simulink model "UAV_sync_known_sim_wrong_version"  (R2018b)
settings: Solver=ode23tb  StartTime=0.0  StopTime=35
values from neighbouring files (symbols this model uses):
  C_rho = 1.225    [SC42120_UAV_Preconditions.m]
  D0 = [M0 0 0 0 0 0 ... (first row only)    [SC42120_UAV_Preconditions.m]
  D1 = [eye(3)*M1 zeros(3,3) ... (first row only)    [UAV_sync_known.m]    (also in UAV_sync_unknown.m; UAV_sync_unknown_gap.m)
  D2 = [eye(3)*M2 zeros(3,3) ... (first row only)    [UAV_sync_known.m]    (also in UAV_sync_unknown.m; UAV_sync_unknown_gap.m)
  Derivative_gain_phi = 50    [SC42120_UAV_Preconditions.m]
  Derivative_gain_psi = 50    [SC42120_UAV_Preconditions.m]
  Derivative_gain_theta = 50    [SC42120_UAV_Preconditions.m]
  Derivative_gain_x = 50    [SC42120_UAV_Preconditions.m]
  Derivative_gain_y = 50    [SC42120_UAV_Preconditions.m]
  Derivative_gain_z = 50    [SC42120_UAV_Preconditions.m]
  G = 9.80665    [SC42120_UAV_Preconditions.m]
  g0 = [0;0;-M0*G;0;0;0]    [SC42120_UAV_Preconditions.m]
  I0 = [0.02 0 -0.01 ... (first row only)    [SC42120_UAV_Preconditions.m]
  I1 = [0.1 0 -0.01 ... (first row only)    [UAV_sync_known.m]    (also in UAV_sync_unknown.m; UAV_sync_unknown_gap.m)
  I2 = 2*[0.1 0 -0.01 ... (first row only)    [UAV_sync_known.m]    (also in UAV_sync_unknown.m; UAV_sync_unknown_gap.m)
  InitWind = [0;0;0]    [SC42120_UAV_Preconditions.m]
  Kp = diag(P)    [SC42120_UAV_Preconditions.m]
  Kv = diag(V)    [SC42120_UAV_Preconditions.m]
  M0 = 10    [SC42120_UAV_Preconditions.m]
  M1 = 20    [UAV_sync_known.m]    (also in UAV_sync_unknown.m; UAV_sync_unknown_gap.m)
  M2 = 30    [UAV_sync_known.m]    (also in UAV_sync_unknown.m; UAV_sync_unknown_gap.m)
  Proportional_phi = 50    [SC42120_UAV_Preconditions.m]
  Proportional_psi = 50    [SC42120_UAV_Preconditions.m]
  Proportional_theta = 50    [SC42120_UAV_Preconditions.m]
  Proportional_x = 50    [SC42120_UAV_Preconditions.m]
  Proportional_y = 50    [SC42120_UAV_Preconditions.m]
  Proportional_z = 50    [SC42120_UAV_Preconditions.m]
undefined symbols (not defined in the file or in its folder): Aero, APlane, Bxl, C, Ctr, deg, DiscIntNeverNeededParam, F, Guid, Init, Light, MIL, Path, rad, s, Trim, Utility
libraries: aerolibconvert2 x37, simulink x15, dspsigops x7, shared6dof x4, aerolibasang x4, sharedutil x4, simulink_extras x3, aerolibadyn x1, aerolibtransform2 x1, aerolibwind2 x1
(part 5 of 6)

== system UAV_sync_known_sim_wrong_version/Node 0/VF Approach/BIXLER DYNAMICS/Vehicle Airframe/Aerodynamics/Forces//Moments ==
  note: From stability frame to body frame
  CD : Inport
  Cy : Inport  Port=2
  CL : Inport  Port=3
  Cl : Inport  Port=4
  Cm : Inport  Port=5
  Cn : Inport  Port=6
  DerCond : Inport  Port=7
  "Aerodynamic Forces and Moments " : aerolibadyn/Aerodynamic Forces and Moments   inputAxes=Body  outputForceAxes=Body  outputMomentAxes=Body  S=Bxl.S  b=Bxl.c  cbar=Bxl.b
      settings: SourceProductName=Aerospace Blockset
  Bus Selector : BusSelector  OutputSignals=qbar
  Constant : Constant  Value=Bxl.COG
  Demux : Demux  Outputs=3
  From wind to body : Math  Operator=transpose  SaturateOnIntegerOverflow=on
  Gain2 : Gain  Gain=-1
  Gain3 : Gain  Gain=-1
  Manual Switch : ManualSwitch  CurrentSetting=0
  Mux : Mux  Inputs=6
  Mux1 : Mux  Inputs=3
  Mux3 : Mux  Inputs=2
  Product : Product  Inputs=**  Multiplication=Matrix(*)
  Rotation Matrix Body to Wind : aerolibtransform2/Direction Cosine Matrix Body to Wind
      settings: SourceProductName=Aerospace Blockset  SourceProductBaseCode=AE
  beta : Constant  Value=0
  neglect center of gravity and center of pressure effects : Constant  Value=[0 0 0]
  Fxyz : Outport
  Mlmn : Outport  Port=2
  wires:
  Demux/1 -> Mux/1  "Cx"
  Demux/3 -> Mux/3  "Cz"
  Mux/1 -> "Aerodynamic Forces and Moments "/1
  Cn/1 -> Mux/6
  CD/1 -> Gain2/1
  Cl/1 -> Mux/4
  Mux1/1 -> Product/2
  Constant/1 -> Manual Switch/1
  "Aerodynamic Forces and Moments "/2 -> Mlmn/1
  "Aerodynamic Forces and Moments "/1 -> Fxyz/1
  Bus Selector/1 -> "Aerodynamic Forces and Moments "/2  "<qbar>"
  DerCond/1 -> Bus Selector/1
  CL/1 -> Gain3/1
  Cm/1 -> Mux/5
  [alphaRad] -> Mux3/1
  beta/1 -> Mux3/2
  Mux3/1 -> Rotation Matrix Body to Wind/1
  Rotation Matrix Body to Wind/1 -> From wind to body/1
  Gain2/1 -> Mux1/1
  Gain3/1 -> Mux1/3
  Cy/1 -> Mux1/2
  From wind to body/1 -> Product/1
  Product/1 -> Demux/1
  Demux/2 -> Mux/2  "Cy"
  neglect center of gravity and center of pressure effects/1 -> Manual Switch/2
  Manual Switch/1 -> "Aerodynamic Forces and Moments "/4, "Aerodynamic Forces and Moments "/3

== system UAV_sync_known_sim_wrong_version/Node 0/VF Approach/BIXLER DYNAMICS/Vehicle Airframe/Propulsion/By interpolation ==
  In1 : Inport
  Prelookup : PreLookup  BreakpointsData=Aero.thrust_vect  BeginIndexSearchUsingPreviousIndexResult=on  RemoveProtectionInput=on
  Throttle interpolation : Interpolation_n-D  NumberOfTableDimensions=1  Table=Aero.thrust_force_vect  ExtrapMethod=Clip  RemoveProtectionIndex=on  InternalRulePriority=Speed
      settings: InputPortMap=u0,u1
  Out1 : Outport
  wires:
  Prelookup/1 -> Throttle interpolation/1
  Prelookup/2 -> Throttle interpolation/2
  Throttle interpolation/1 -> Out1/1
  In1/1 -> Prelookup/1

== system UAV_sync_known_sim_wrong_version/Node 0/VF Approach/BIXLER DYNAMICS/Vehicle Airframe/Propulsion/Propeller model (Bernoulli) ==
  DerCond : Inport
  Throttle : Inport  Port=2
  0.5 * C.rho * Bxl.S_prop * Bxl.rotor_thrust_coeff : Gain  Gain=0.5 * C.rho * Bxl.S_prop * Bxl.rotor_thrust_coeff
  Bus Selector : BusSelector  OutputSignals=Va
  Bxl.r_prop : Gain  Gain=Bxl.r_prop*0.5
  Math Function : Math  Operator=square  SaturateOnIntegerOverflow=on
  Math Function1 : Math  Operator=square  SaturateOnIntegerOverflow=on
  Sum : Sum  Inputs=+-
  k_motor * u + q_motor : Fcn  Expr=Bxl.k_motor * u + Bxl.q_motor
  Thrust : Outport
  wires:
  Math Function/1 -> Sum/2  "V_a^2"
  Sum/1 -> 0.5 * C.rho * Bxl.S_prop * Bxl.rotor_thrust_coeff/1
  DerCond/1 -> Bus Selector/1
  Throttle/1 -> k_motor * u + q_motor/1
  0.5 * C.rho * Bxl.S_prop * Bxl.rotor_thrust_coeff/1 -> Thrust/1  "T"
  Bxl.r_prop/1 -> Math Function1/1  "Air flow velocity after prop."
  k_motor * u + q_motor/1 -> Bxl.r_prop/1  "Prop. angular speed (Omega)"
  Math Function1/1 -> Sum/1  "(R*Ome)^2"
  Bus Selector/1 -> Math Function/1  "<Va>"

== system UAV_sync_known_sim_wrong_version/Node 0/VF Approach/PATH FOLLOWING/Orbit Path Following (Enabled Subsystem)/Chi_d/While Iterator Subsystem ==
  gamma : Inport
  chi : Inport  Port=2
  IC : Inport  Port=3
  Bias : Bias  Bias=2*pi
  Constant : Constant  Value=-pi
  Relational Operator : RelationalOperator  Operator=<  OutDataTypeStr=boolean  RndMeth=Simplest
  Sum : Sum  Inputs=|+-
  While Iterator : WhileIterator  ResetStates=reset
  gaooa_out : Outport
  wires:
  IC/1 -> While Iterator/2
  gamma/1 -> Bias/1, Sum/1
  chi/1 -> Sum/2
  Sum/1 -> Relational Operator/1
  Constant/1 -> Relational Operator/2
  Relational Operator/1 -> While Iterator/1
  Bias/1 -> gaooa_out/1

== system UAV_sync_known_sim_wrong_version/Node 0/VF Approach/PATH FOLLOWING/Orbit Path Following (Enabled Subsystem)/Chi_d/While Iterator Subsystem2 ==
  gamma : Inport
  chi : Inport  Port=2
  IC : Inport  Port=3
  Bias : Bias  Bias=2*pi
  Constant : Constant  Value=pi
  Relational Operator : RelationalOperator  Operator=>  OutDataTypeStr=boolean  RndMeth=Simplest
  Sum : Sum  Inputs=|+-
  While Iterator : WhileIterator  ResetStates=reset
  gaooa_out : Outport
  wires:
  Bias/1 -> gaooa_out/1
  Relational Operator/1 -> While Iterator/1
  Constant/1 -> Relational Operator/2
  Sum/1 -> Relational Operator/1
  chi/1 -> Sum/2
  gamma/1 -> Sum/1, Bias/1
  IC/1 -> While Iterator/2

== system UAV_sync_known_sim_wrong_version/Node 0/VF Approach/PATH FOLLOWING/Orbit Path Following (Enabled Subsystem)/Loiter Controller/Parameters Mixer ==
  Constant1 : Constant  Value=Guid.Est.alpha
  Constant6 : Constant  Value=Guid.Loiter.k
  Constant7 : Constant  Value=Guid.Loiter.kk
  Constant8 : Constant  Value=Guid.Loiter.eps
  Mux : Mux  Inputs=6
  param : Outport
  wires:
  Mux/1 -> param/1
  Constant6/1 -> Mux/1
  Constant7/1 -> Mux/2
  Constant8/1 -> Mux/3
  [R] -> Mux/4
  [j] -> Mux/5
  Constant1/1 -> Mux/6

== system UAV_sync_known_sim_wrong_version/Node 0/VF Approach/PATH FOLLOWING/Orbit Path Following (Enabled Subsystem)/Vg Estimator/Parameters Mixer ==
  airspeed : Inport
  Constant : Constant  Value=Guid.Wind.W
  Constant1 : Constant  Value=Guid.Wind.phiw
  Constant11 : Constant  Value=Guid.Loiter.gamma
  Constant2 : Constant  Value=Guid.Loiter.d_int
  Constant3 : Constant  Value=Guid.Loiter.sigma
  Constant6 : Constant  Value=Guid.Loiter.k
  Constant7 : Constant  Value=Guid.Loiter.kk
  Constant8 : Constant  Value=Guid.Loiter.eps
  From27 : From  Commented=on  GotoTag=Target_Airspeed  TagVisibility=global
  Mux : Mux  Inputs=11
  param : Outport
  wires:
  Constant11/1 -> Mux/10
  [R] -> Mux/8
  Mux/1 -> param/1
  [j] -> Mux/9
  Constant/1 -> Mux/1
  Constant8/1 -> Mux/6
  Constant6/1 -> Mux/4
  Constant7/1 -> Mux/5
  airspeed/1 -> Mux/3
  Constant1/1 -> Mux/2
  Constant2/1 -> Mux/7
  Constant3/1 -> Mux/11

== system UAV_sync_known_sim_wrong_version/Node 0/VF Approach/PATH FOLLOWING/Straight-line Path Following (Enabled Subsystem)/SL.controller/Param. Mixer ==
  Constant1 : Constant  Value=Guid.SL.chi_inf
  Constant2 : Constant  Value=Guid.Est.alpha
  Constant3 : Constant  Value=Guid.SL.kk
  Constant4 : Constant  Value=Guid.SL.eps
  Constant5 : Constant  Value=Guid.SL.k
  Mux : Mux  Inputs=5
  param : Outport
  wires:
  Constant2/1 -> Mux/5  "alpha"
  Constant3/1 -> Mux/4  "kk"
  Constant5/1 -> Mux/3  "k"
  Constant1/1 -> Mux/2  "chi_inf"
  Constant4/1 -> Mux/1  "eps"
  Mux/1 -> param/1

== system UAV_sync_known_sim_wrong_version/Node 0/VF Approach/PATH FOLLOWING/Straight-line Path Following (Enabled Subsystem)/Vg Estimator/Param. Mixer ==
  Va : Inport
  Constant1 : Constant  Value=Guid.Wind.W
  Constant12 : Constant  Value=Guid.SL.gamma
  Constant2 : Constant  Value=Guid.Wind.phiw
  Constant3 : Constant  Value=Guid.SL.eps
  Constant4 : Constant  Value=Guid.SL.epy
  Constant5 : Constant  Value=Guid.SL.sigma
  Constant6 : Constant  Value=Guid.SL.chi_inf
  Constant7 : Constant  Value=Guid.SL.k
  Constant8 : Constant  Value=Guid.SL.kk
  Constant9 : Constant  Value=Guid.Est.alpha
  Mux : Mux  Inputs=11
  param : Outport
  wires:
  Mux/1 -> param/1
  Constant4/1 -> Mux/1  "y_int"
  Constant6/1 -> Mux/6  "chi_inf"
  Constant7/1 -> Mux/7  "k"
  Constant1/1 -> Mux/2  "W"
  Constant8/1 -> Mux/8  "kk"
  Constant3/1 -> Mux/4  "epsilon"
  Constant2/1 -> Mux/5  "phiw = constant wind direction"
  Constant12/1 -> Mux/9  "gamma"
  Constant5/1 -> Mux/10  "sigma"
  Va/1 -> Mux/3  "Va"
  Constant9/1 -> Mux/11  "alpha"

== system UAV_sync_known_sim_wrong_version/Node 0/VF Approach/AUTOPILOT/Low-level Controllers/Pitch controller/Coordination offset/cos ==
  In1 : Inport
  Trigonometric Function : Trigonometry  Operator=cos
  Out1 : Outport
  wires:
  In1/1 -> Trigonometric Function/1
  Trigonometric Function/1 -> Out1/1

== system UAV_sync_known_sim_wrong_version/Node 0/VF Approach/AUTOPILOT/Low-level Controllers/Pitch controller/Coordination offset/sin ==
  In1 : Inport
  Angle Conversion : aerolibconvert2/Angle Conversion  Commented=through  IU=deg  OU=rad
  Angle Conversion1 : aerolibconvert2/Angle Conversion  Commented=through  IU=rad  OU=deg
  Trigonometric Function : Trigonometry
  Out1 : Outport
  wires:
  Trigonometric Function/1 -> Angle Conversion1/1
  Angle Conversion/1 -> Trigonometric Function/1
  Angle Conversion1/1 -> Out1/1
  In1/1 -> Angle Conversion/1

== system UAV_sync_known_sim_wrong_version/Node 0/VF Approach/AUTOPILOT/Low-level Controllers/Pitch controller/Coordination offset/tan ==
  In1 : Inport
  Angle Conversion : aerolibconvert2/Angle Conversion  Commented=through  IU=deg  OU=rad
  Angle Conversion1 : aerolibconvert2/Angle Conversion  Commented=through  IU=rad  OU=deg
  Trigonometric Function : Trigonometry  Operator=tan
  Out1 : Outport
  wires:
  In1/1 -> Angle Conversion/1
  Angle Conversion1/1 -> Out1/1
  Angle Conversion/1 -> Trigonometric Function/1
  Trigonometric Function/1 -> Angle Conversion1/1

== system UAV_sync_known_sim_wrong_version/Node 0/VF Approach/AUTOPILOT/Low-level Controllers/Pitch controller/Pitch PID/Adjust integrator gain ==
  Constant10 : Constant  Value=0.15
  Ctr.Pitch.PTCH2SRV_TCONST : Gain  Gain=Ctr.Pitch.PTCH2SRV_TCONST
  MinMax : MinMax  Function=max  Inputs=2
  K_I rate : Outport
  wires:
  ? -> MinMax/1
  Ctr.Pitch.PTCH2SRV_TCONST/1 -> K_I rate/1  "ki_rate"
  Constant10/1 -> MinMax/2
  MinMax/1 -> Ctr.Pitch.PTCH2SRV_TCONST/1

== system UAV_sync_known_sim_wrong_version/Node 0/VF Approach/AUTOPILOT/Low-level Controllers/Pitch controller/Pitch PID/Anti-windup ==
  u : Inport
  y : Inport  Port=2
  If : If  IfExpression=u1 < -45  ElseIfExpressions=u1 > 45
  If Action Subsystem : Subsystem  TreatAsAtomicUnit=on
  If Action Subsystem1 : Subsystem  TreatAsAtomicUnit=on
  If Action Subsystem2 : Subsystem  TreatAsAtomicUnit=on
  Merge : Merge  Inputs=3
  y_int : Outport
  wires:
  If Action Subsystem1/1(Out1) -> Merge/2
  Merge/1 -> y_int/1
  If Action Subsystem2/1(Out1) -> Merge/3
  y/1 -> If/1
  If Action Subsystem/1(Out1) -> Merge/1
  u/1 -> If Action Subsystem/1(In1), If Action Subsystem1/1(In1), If Action Subsystem2/1(In1)
  If/2 -> If Action Subsystem1/Action
  If/1 -> If Action Subsystem/Action
  If/3 -> If Action Subsystem2/Action

== system UAV_sync_known_sim_wrong_version/Node 0/VF Approach/AUTOPILOT/Low-level Controllers/Pitch controller/Pitch PID/Subsystem ==
  In1 : Inport
  Meas_roll_angle : Inport  Port=2
  Meas_pitch_rate : Inport  Port=3  Unit=deg/s
  +-45 : Saturate  UpperLimit=45  LowerLimit=-45
  Abs : Abs
  Abs1 : Abs
  Gain : Gain  Gain=-1
  If : If  IfExpression=u1 > 90
  If Action Subsystem : Subsystem  TreatAsAtomicUnit=on
  If Action Subsystem1 : Subsystem  TreatAsAtomicUnit=on
  If Action Subsystem2 : Subsystem  TreatAsAtomicUnit=on
  If Action Subsystem3 : Subsystem  TreatAsAtomicUnit=on
  If1 : If  NumInputs=2  IfExpression=u1 >84 & u2 < 70
  Merge : Merge
  Merge1 : Merge
  Out1 : Outport
  wires:
  If Action Subsystem3/1(Out1) -> Merge1/2
  Abs/1 -> If Action Subsystem/1(In1), If Action Subsystem1/1(In1), If/1
  Meas_pitch_rate/1 -> Abs1/1
  If/1 -> If Action Subsystem/Action
  Merge/1 -> If Action Subsystem2/1(In1), If1/1  "roll wrapped"
  If Action Subsystem2/1(Out1) -> Merge1/1
  +-45/1 -> Gain/1
  If1/2 -> If Action Subsystem3/Action
  Abs1/1 -> If1/2
  If Action Subsystem1/1(Out1) -> Merge/2
  Meas_roll_angle/1 -> Abs/1
  If1/1 -> If Action Subsystem2/Action
  In1/1 -> If Action Subsystem3/1(In1), If Action Subsystem2/2(In2)
  Gain/1 -> Out1/1
  If Action Subsystem/1(Out1) -> Merge/1
  If/2 -> If Action Subsystem1/Action
  Merge1/1 -> [lastO], +-45/1

== system UAV_sync_known_sim_wrong_version/Node 0/VF Approach/AUTOPILOT/Low-level Controllers/Pitch controller/TRASH/If Action Subsystem ==
  Action Port : ActionPort
  Constant : Constant  Value=0
  Out1 : Outport
  wires:
  Constant/1 -> Out1/1

== system UAV_sync_known_sim_wrong_version/Node 0/VF Approach/AUTOPILOT/Low-level Controllers/Pitch controller/TRASH/If Action Subsystem1 ==
  pitch : Inport
  bank : Inport  Port=2
  Va : Inport  Port=3
  Action Port : ActionPort
  Abs : Abs
  Constant : Constant  Value=C.g
  Constant1 : Constant  Value=APlane.EAS2TAS
  Constant2 : Constant  Value=APlane.airspeed_min
  Constant3 : Constant  Value=Ctr.Pitch.PTCH2SRV_RLL
  MinMax : MinMax  Function=max  Inputs=2
  Product : Product  Inputs=***
  Product1 : Product  Inputs=*/**
  Product2 : Product  Inputs=**
  bank1 : InportShadow  Port=2
  cosd : Subsystem
  sind : Subsystem
  tand : Subsystem
  Out1 : Outport
  wires:
  Product/1 -> Out1/1
  Abs/1 -> Product/2
  Constant/1 -> Product1/1
  MinMax/1 -> Product1/2
  Constant1/1 -> Product2/2
  Va/1 -> Product2/1
  Product2/1 -> MinMax/1
  Constant2/1 -> MinMax/2
  cosd/1(Out1) -> Product/1
  bank/1 -> tand/1(In1)
  bank1/1 -> sind/1(In1)
  Product1/1 -> Abs/1
  pitch/1 -> cosd/1(In1)
  tand/1(Out1) -> Product1/3
  sind/1(Out1) -> Product1/4
  Constant3/1 -> Product/3

== system UAV_sync_known_sim_wrong_version/Node 0/VF Approach/AUTOPILOT/Low-level Controllers/Pitch controller/TRASH/Parameters mixer1 ==
  note: 9
  note: 8
  note: 7
  note: 6
  note: 5
  note: 4
  note: 3
  note: 2
  note: 1
  Constant : Constant  Value=Ctr.Pitch.PTCH2SRV_I
  Constant1 : Constant  Value=Ctr.Pitch.PTCH2SRV_D
  Constant2 : Constant  Value=Ctr.Pitch.PTCH2SRV_FF
  Constant3 : Constant  Value=Ctr.Pitch.PTCH2SRV_P
  Constant4 : Constant  Value=APlane.roll_limit
  Constant5 : Constant  Value=Ctr.Pitch.PTCH2SRV_IMAX
  Constant6 : Constant  Value=APlane.airspeed_min
  Constant7 : Constant  Value=APlane.EAS2TAS
  Constant8 : Constant  Value=Ctr.Pitch.PTCH2SRV_TCONST
  Mux : Mux  Inputs=9
  parameters : Outport
  wires:
  Mux/1 -> parameters/1
  Constant8/1 -> Mux/1
  Constant3/1 -> Mux/2
  Constant/1 -> Mux/3
  Constant1/1 -> Mux/4
  Constant5/1 -> Mux/5
  Constant2/1 -> Mux/6
  Constant6/1 -> Mux/7
  Constant7/1 -> Mux/8
  Constant4/1 -> Mux/9

== system UAV_sync_known_sim_wrong_version/Node 0/VF Approach/AUTOPILOT/Low-level Controllers/Pitch controller/TRASH/Parameters mixer2 ==
  Constant2 : Constant  Value=Ctr.Pitch.PTCH2SRV_RLL
  Constant3 : Constant  Value=C.g
  Constant5 : Constant  Value=APlane.EAS2TAS
  Constant6 : Constant  Value=APlane.airspeed_min
  Mux1 : Mux
  parameters_roll_comp : Outport
  wires:
  Constant6/1 -> Mux1/4
  Constant5/1 -> Mux1/3
  Mux1/1 -> parameters_roll_comp/1
  Constant3/1 -> Mux1/2
  Constant2/1 -> Mux1/1

== system UAV_sync_known_sim_wrong_version/Node 0/VF Approach/AUTOPILOT/Low-level Controllers/Roll controller/Roll Rate Controller/Anti-windup ==
  y : Inport
  u : Inport  Port=2
  If : If  IfExpression=u1 < -45  ElseIfExpressions=u1 > 45
  If Action Subsystem : Subsystem  TreatAsAtomicUnit=on
  If Action Subsystem1 : Subsystem  TreatAsAtomicUnit=on
  If Action Subsystem2 : Subsystem  TreatAsAtomicUnit=on
  Merge : Merge  Inputs=3
  y_int : Outport
  wires:
  If Action Subsystem1/1(Out1) -> Merge/2
  Merge/1 -> y_int/1
  If Action Subsystem2/1(Out1) -> Merge/3
  y/1 -> If/1
  If Action Subsystem/1(Out1) -> Merge/1
  u/1 -> If Action Subsystem/1(In1), If Action Subsystem1/1(In1), If Action Subsystem2/1(In1)
  If/2 -> If Action Subsystem1/Action
  If/1 -> If Action Subsystem/Action
  If/3 -> If Action Subsystem2/Action

== system UAV_sync_known_sim_wrong_version/Node 0/VF Approach/AUTOPILOT/Low-level Controllers/Roll controller/Roll Rate Controller/K_FF (real feedforward) ==
  Constant5 : Constant  Value=Ctr.Roll.RLL2SRV_FF
  Constant6 : Constant  Value=APlane.EAS2TAS
  Product1 : Product  Inputs=*/
  Out1 : Outport
  wires:
  Product1/1 -> Out1/1  "k_ff"
  Constant6/1 -> Product1/2
  Constant5/1 -> Product1/1

== system UAV_sync_known_sim_wrong_version/Node 0/VF Approach/AUTOPILOT/Low-level Controllers/Roll controller/Roll Rate Controller/K_P (feedforward) ==
  Constant : Constant  Value=APlane.EAS2TAS
  Constant2 : Constant  Value=0
  Constant7 : Constant  Value=Ctr.Roll.K_P
  MinMax : MinMax  Function=max  Inputs=2
  Product : Product  Inputs=*/
  Out1 : Outport
  wires:
  Constant2/1 -> MinMax/2
  Constant7/1 -> MinMax/1
  MinMax/1 -> Product/1
  Product/1 -> Out1/1  "kp_ff"
  Constant/1 -> Product/2

== system UAV_sync_known_sim_wrong_version/Node 0/VF Approach/BIXLER DYNAMICS/RUBBISH BIN/Straight Line/SL.controller/Param. Mixer ==
  Constant1 : Constant  Value=Guid.SL.chi_inf
  Constant2 : Constant  Value=Guid.Est.alpha
  Constant3 : Constant  Value=Guid.SL.kk
  Constant4 : Constant  Value=Guid.SL.eps
  Constant5 : Constant  Value=Guid.SL.k
  Mux : Mux  Inputs=5
  param : Outport
  wires:
  Constant2/1 -> Mux/5  "alpha"
  Constant3/1 -> Mux/4  "kk"
  Constant5/1 -> Mux/3  "k"
  Constant1/1 -> Mux/2  "chi_inf"
  Constant4/1 -> Mux/1  "eps"
  Mux/1 -> param/1

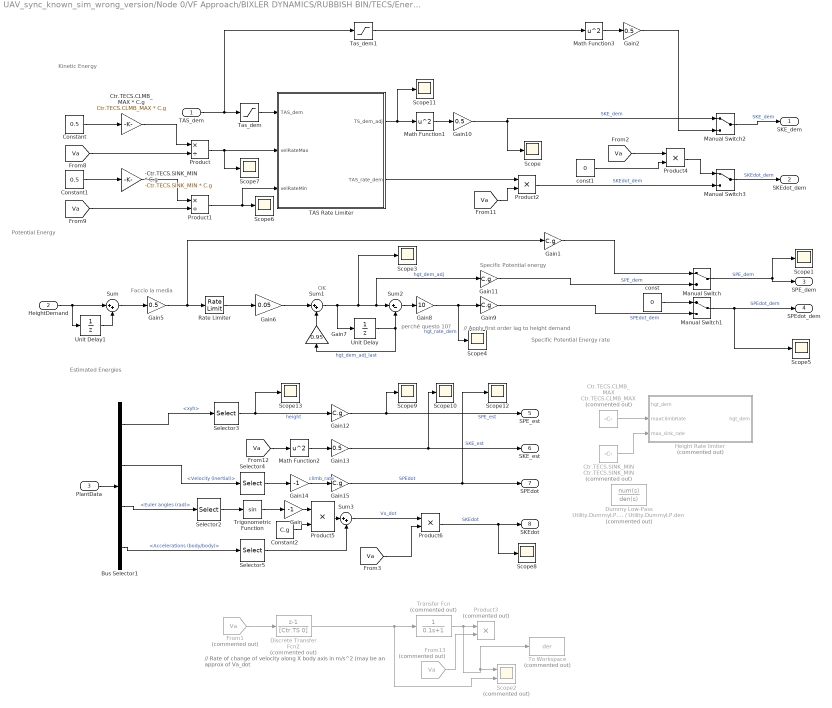
== system UAV_sync_known_sim_wrong_version/Node 0/VF Approach/BIXLER DYNAMICS/RUBBISH BIN/TECS/Energy calculations/Calculate energies ==
  note: Estimated Energies
  note: Potential Energy
  note: Kinetic Energy
  note: // Apply first order lag to height demand
  note: perché questo 10?
  note: Specific Potential Energy rate
  note: Specific Potential energy
  note: OK
  note: Faccio la media
  note: // Rate of change of velocity along X body axis in m/s^2
      | (may be an approx of Va_dot
  TAS_dem : Inport
  HeightDemand : Inport  Port=2
  PlantData : Inport  Port=3
  -Ctr.TECS.SINK_MIN * C.g : Gain  Gain=-Ctr.TECS.SINK_MIN * C.g
  Bus Selector1 : BusSelector  OutputSignals=xyh,Velocity (inertial),Euler angles (rad),Accelerations (body/body)
  Constant : Constant  Value=0.5
  Constant1 : Constant  Value=0.5
  Constant2 : Constant  Value=C.g
  Ctr.TECS.CLMB_MAX : Constant  Commented=on  Value=Ctr.TECS.CLMB_MAX
  Ctr.TECS.CLMB_MAX * C.g : Gain  Gain=Ctr.TECS.CLMB_MAX * C.g
  Ctr.TECS.SINK_MIN : Constant  Commented=on  Value=Ctr.TECS.SINK_MIN
  Discrete Transfer Fcn2 : DiscreteTransferFcn  Commented=on  Numerator=[1 -1]  Denominator=[Ctr.TS 0]  SampleTime=Ctr.TS
  Dummy Low-Pass : TransferFcn  Commented=on  Numerator=Utility.DummyLP.num  Denominator=Utility.DummyLP.den
  From1 : From  Commented=on  GotoTag=Va  TagVisibility=global
  From13 : From  Commented=on  GotoTag=Va  TagVisibility=global
  Gain : Gain  Gain=-1
  Gain{1,9,11..12,15} (5 alike) : Gain  Gain=C.g
  Gain{2,5,10,13} (4 alike) : Gain  Gain=0.5
  Gain14 : Gain  Gain=-1
  Gain6 : Gain  Gain=0.05
  Gain7 : Gain  Gain=0.95
  Gain8 : Gain  Gain=10
  Height Rate limiter : MATLAB Function  Commented=on  TreatAsAtomicUnit=on
  Manual Switch{,1..3} (4 alike) : ManualSwitch
  Math Function1 : Math  Operator=square  SaturateOnIntegerOverflow=on
  Math Function2 : Math  Operator=square  SaturateOnIntegerOverflow=on
  Math Function3 : Math  Operator=square  SaturateOnIntegerOverflow=on
  Product : Product  Inputs=*/
  Product1 : Product  Inputs=*/
  Product{2,4..6} (4 alike) : Product
  Product3 : Product  Commented=on
  Rate Limiter : RateLimiter  RisingSlewLimit=Ctr.TECS.CLMB_MAX  FallingSlewLimit=-Ctr.TECS.SINK_MIN  SampleTimeMode=inherited
  Scope{,1,3..13} (13 alike) : Scope
  Scope2 : Scope  Commented=on  NumInputPorts=2
  Selector2 : Selector  InputPortWidth=3  IndexOptions=Index vector (dialog)  Indices=2  OutputSizes=1
  Selector3 : Selector  InputPortWidth=3  IndexOptions=Index vector (dialog)  Indices=3  OutputSizes=1
  Selector4 : Selector  InputPortWidth=3  IndexOptions=Index vector (dialog)  Indices=3  OutputSizes=1
  Selector5 : Selector  InputPortWidth=3  IndexOptions=Index vector (dialog)  Indices=1  OutputSizes=1
  Sum : Sum  Inputs=|++
  Sum1 : Sum  Inputs=|++
  Sum2 : Sum  Inputs=|+-
  Sum3 : Sum  Inputs=|++
  TAS Rate Limiter : MATLAB Function  TreatAsAtomicUnit=on
  Tas_dem : Saturate  UpperLimit=35  LowerLimit=6
  Tas_dem1 : Saturate  UpperLimit=35  LowerLimit=6
  To Workspace : ToWorkspace  Commented=on  VariableName=der  SampleTime=-1
  Transfer Fcn : TransferFcn  Commented=on  Numerator=1  Denominator=[0.1 1]
  Trigonometric Function : Trigonometry
  Unit Delay : UnitDelay  SampleTime=Ctr.TS
  Unit Delay1 : UnitDelay  SampleTime=Ctr.TS
  const : Constant  Value=0
  const1 : Constant  Value=0
  SKE_dem : Outport
  SKEdot_dem : Outport  Port=2
  SPE_dem : Outport  Port=3
  SPEdot_dem : Outport  Port=4
  SPE_est : Outport  Port=5
  SKE_est : Outport  Port=6
  SPEdot : Outport  Port=7
  SKEdot : Outport  Port=8
  wires:
  Gain5/1 -> Gain1/1, Rate Limiter/1
  Gain8/1 -> Scope4/1, Gain9/1  "hgt_rate_dem"
  Gain6/1 -> Sum1/1
  Sum/1 -> Gain5/1
  Ctr.TECS.CLMB_MAX/1 -> Height Rate limiter/2(maxClimbRate)
  Ctr.TECS.SINK_MIN/1 -> Height Rate limiter/3(max_sink_rate)
  -Ctr.TECS.SINK_MIN * C.g/1 -> Product1/1
  Ctr.TECS.CLMB_MAX * C.g/1 -> Product/1
  Manual Switch/1 -> SPE_dem/1, Scope1/1  "SPE_dem"
  Sum2/1 -> Gain8/1
  Unit Delay/1 -> Gain7/1, Sum2/2  "hgt_dem_adj_last"
  Product2/1 -> Manual Switch3/2  "SKEdot_dem"
  Sum1/1 -> Unit Delay/1, Scope3/1, Gain11/1, Sum2/1  "hgt_dem_adj"
  Manual Switch1/1 -> Scope5/1, SPEdot_dem/1  "SPEdot_dem"
  [Va] -> Product2/2
  Gain12/1 -> Scope9/1, SPE_est/1  "SPE_est"
  Gain14/1 -> Gain15/1  "climb_rate"
  Gain13/1 -> Scope10/1, SKE_est/1  "SKE_est"
  TAS Rate Limiter/1(TS_dem_adj) -> Scope11/1, Math Function1/1
  Math Function2/1 -> Gain13/1
  TAS Rate Limiter/2(TAS_rate_dem) -> Product2/1
  Gain10/1 -> Manual Switch2/1, Scope/1  "SKE_dem"
  Math Function1/1 -> Gain10/1
  Selector3/1 -> Scope13/1, Gain12/1  "height"
  [Va] -> Math Function2/1
  Constant1/1 -> -Ctr.TECS.SINK_MIN * C.g/1
  Product1/1 -> Scope6/1, TAS Rate Limiter/3(velRateMin)
  Product/1 -> Scope7/1, TAS Rate Limiter/2(velRateMax)
  Gain7/1 -> Sum1/2
  Constant/1 -> Ctr.TECS.CLMB_MAX * C.g/1
  TAS_dem/1 -> Tas_dem1/1, Tas_dem/1
  HeightDemand/1 -> Unit Delay1/1, Sum/1
  Gain15/1 -> Scope12/1, SPEdot/1  "SPEdot"
  PlantData/1 -> Bus Selector1/1
  Bus Selector1/1 -> Selector3/1  "<xyh>"
  Bus Selector1/2 -> Selector4/1  "<Velocity (inertial)>"
  [Va] -> Product/2
  Selector4/1 -> Gain14/1
  [Va] -> Product1/2
  Rate Limiter/1 -> Gain6/1
  Unit Delay1/1 -> Sum/2
  Gain11/1 -> Manual Switch/2  "SPE_dem"
  Gain9/1 -> Manual Switch1/2  "SPEdot_dem"
  Gain1/1 -> Manual Switch/1
  Manual Switch2/1 -> SKE_dem/1  "SKE_dem"
  Math Function3/1 -> Gain2/1
  Gain2/1 -> Manual Switch2/2
  const1/1 -> Product4/2
  Tas_dem/1 -> TAS Rate Limiter/1(TAS_dem)
  [Va] -> Product4/1
  Product4/1 -> Manual Switch3/1
  Manual Switch3/1 -> SKEdot_dem/1  "SKEdot_dem"
  From13/1 -> Product3/2
  Product6/1 -> Scope8/1, SKEdot/1  "SKEdot"
  From1/1 -> Discrete Transfer Fcn2/1
  Discrete Transfer Fcn2/1 -> Transfer Fcn/1, Scope2/2
  Transfer Fcn/1 -> To Workspace/1, Scope2/1, Product3/1
  Bus Selector1/3 -> Selector2/1  "<Euler angles (rad)>"
  Sum3/1 -> Product6/1  "Vx_dot"
  [Va] -> Product6/2
  Selector2/1 -> Trigonometric Function/1
  Constant2/1 -> Product5/2
  Bus Selector1/4 -> Selector5/1  "<Accelerations (body/body)>"
  Product5/1 -> Sum3/1
  Selector5/1 -> Sum3/2
  Gain/1 -> Product5/1
  Trigonometric Function/1 -> Gain/1
  Tas_dem1/1 -> Math Function3/1
  const/1 -> Manual Switch1/1

== system UAV_sync_known_sim_wrong_version/Node 0/VF Approach/BIXLER DYNAMICS/RUBBISH BIN/TECS/PITCH/DT1 ==
  Clock1 : Clock
  Memory : Memory  InheritSampleTime=on
  Sum : Sum  Inputs=|+-
  DT : Outport
  wires:
  Memory/1 -> Sum/2
  Sum/1 -> DT/1
  Clock1/1 -> Memory/1, Sum/1

== system UAV_sync_known_sim_wrong_version/Node 0/VF Approach/BIXLER DYNAMICS/RUBBISH BIN/TECS/PITCH/Limiter ==
  integSEB_input : Inport
  PITCHmaxf : Inport  Port=2
  PITCHminf : Inport  Port=3
  pitch_dem : Inport  Port=4
  If : If  NumInputs=3  IfExpression=u1 > u2  ElseIfExpressions=u1 < u3
  If Action Subsystem : Subsystem  TreatAsAtomicUnit=on
  If Action Subsystem1 : Subsystem  TreatAsAtomicUnit=on
  If Action Subsystem2 : Subsystem  TreatAsAtomicUnit=on
  Merge : Merge  Inputs=3
  PITCHmaxf_1 : InportShadow  Port=2
  PITCHminf_1 : InportShadow  Port=3
  pitch_dem_1 : InportShadow  Port=4
  SEB_in_lim : Outport
  wires:
  If Action Subsystem1/1(Out1) -> Merge/3
  If Action Subsystem/1(Out1) -> Merge/1
  If Action Subsystem2/1(Out1) -> Merge/2
  PITCHminf_1/1 -> If Action Subsystem1/2(PITCHminf)
  integSEB_input/1 -> If/1, If Action Subsystem1/1(integSEB_input), If Action Subsystem2/1(integSEB_input), If Action Subsystem/1(integSEB_input)
  pitch_dem_1/1 -> If Action Subsystem1/3(pitch_dem)
  PITCHmaxf_1/1 -> If Action Subsystem/2(PITCHmaxf)
  If/3 -> If Action Subsystem2/Action
  PITCHmaxf/1 -> If/2
  Merge/1 -> SEB_in_lim/1
  PITCHminf/1 -> If/3
  pitch_dem/1 -> If Action Subsystem/3(pitch_dem)
  If/1 -> If Action Subsystem/Action
  If/2 -> If Action Subsystem1/Action

== system UAV_sync_known_sim_wrong_version/Node 0/VF Approach/BIXLER DYNAMICS/RUBBISH BIN/TECS/PITCH/integSEB ==
  temp : Inport
  gainInv : Inport  Port=2
  PITCHminf : Inport  Port=3
  PITCHmaxf : Inport  Port=4
  integSEB_delta : Inport  Port=5
  Constant : Constant  Value=0.0783
  Constant1 : Constant  Value=0.0783
  Gain : Gain  Gain=0.1
  Gain1 : Gain  Gain=-0.1
  Product : Product
  Product1 : Product
  Saturation Dynamic : simulink/Discontinuities/Saturation Dynamic  OutMin=[]  OutMax=[]  OutDataTypeStr=Inherit: Same as second input  OutDataType=fixdt(1, 16)  OutScaling=2^-10  DoSatur=off
  Sum : Sum  Inputs=|+-
  Sum1 : Sum  Inputs=|+-
  Sum2 : Sum  Inputs=|++
  Sum3 : Sum  Inputs=-+|
  Sum4 : Sum  Inputs=|+-
  gainInv_1 : InportShadow  Port=2
  "integSEB_min " : Outport
  "IntegSEB_delta " : Outport  Port=2
  integSEB_max : Outport  Port=3
  wires:
  PITCHminf/1 -> Sum/1
  Product/1 -> Sum1/1
  Constant1/1 -> Sum2/2
  Sum3/1 -> integSEB_max/1, [integSEB_max]
  PITCHmaxf/1 -> Sum2/1
  Sum2/1 -> Product1/2
  gainInv_1/1 -> Product1/1
  Constant/1 -> Sum/2
  integSEB_delta/1 -> Saturation Dynamic/2
  Sum/1 -> Product/2
  Sum1/1 -> "integSEB_min "/1, [integSEB_min]
  temp/1 -> Sum3/1, Sum1/2
  [integSEB_range] -> Gain1/1
  Gain1/1 -> Saturation Dynamic/3
  Saturation Dynamic/1 -> "IntegSEB_delta "/1
  Sum4/1 -> [integSEB_range]
  [integSEB_min] -> Sum4/2
  [integSEB_max] -> Sum4/1
  [integSEB_range] -> Gain/1
  Gain/1 -> Saturation Dynamic/1
  gainInv/1 -> Product/1
  Product1/1 -> Sum3/2

== system UAV_sync_known_sim_wrong_version/Node 0/VF Approach/BIXLER DYNAMICS/RUBBISH BIN/TECS/PITCH/timeConstant() ==
  Constant1 : Constant  Value=0.1
  Constant5 : Constant  Value=Ctr.TECS.TIME_CONST
  MinMax : MinMax  Function=max  Inputs=2
  timeConstant : Outport
  wires:
  MinMax/1 -> timeConstant/1
  Constant1/1 -> MinMax/2
  Constant5/1 -> MinMax/1

== system UAV_sync_known_sim_wrong_version/Node 0/VF Approach/BIXLER DYNAMICS/RUBBISH BIN/TECS/PITCH/timeConstant()1 ==
  Constant1 : Constant  Value=0.1
  Constant5 : Constant  Value=Ctr.TECS.TIME_CONST
  MinMax : MinMax  Function=max  Inputs=2
  timeConstant : Outport
  wires:
  MinMax/1 -> timeConstant/1
  Constant1/1 -> MinMax/2
  Constant5/1 -> MinMax/1

== system UAV_sync_known_sim_wrong_version/Node 0/VF Approach/BIXLER DYNAMICS/RUBBISH BIN/TECS/PITCH1/DT1 ==
  Clock1 : Clock
  Memory : Memory  InheritSampleTime=on
  Sum : Sum  Inputs=|+-
  DT : Outport
  wires:
  Memory/1 -> Sum/2
  Sum/1 -> DT/1
  Clock1/1 -> Memory/1, Sum/1

== system UAV_sync_known_sim_wrong_version/Node 0/VF Approach/BIXLER DYNAMICS/RUBBISH BIN/TECS/PITCH1/Limiter ==
  integSEB_input : Inport
  PITCHmaxf : Inport  Port=2
  PITCHminf : Inport  Port=3
  pitch_dem : Inport  Port=4
  If : If  NumInputs=3  IfExpression=u1 > u2  ElseIfExpressions=u1 < u3
  If Action Subsystem : Subsystem  TreatAsAtomicUnit=on
  If Action Subsystem1 : Subsystem  TreatAsAtomicUnit=on
  If Action Subsystem2 : Subsystem  TreatAsAtomicUnit=on
  Merge : Merge  Inputs=3
  PITCHmaxf_1 : InportShadow  Port=2
  PITCHminf_1 : InportShadow  Port=3
  pitch_dem_1 : InportShadow  Port=4
  y : Outport
  wires:
  If Action Subsystem1/1(Out1) -> Merge/3
  If Action Subsystem/1(Out1) -> Merge/1
  If Action Subsystem2/1(Out1) -> Merge/2
  PITCHminf_1/1 -> If Action Subsystem1/2(PITCHminf)
  integSEB_input/1 -> If/1, If Action Subsystem1/1(integSEB_input), If Action Subsystem2/1(integSEB_input), If Action Subsystem/1(integSEB_input)
  pitch_dem_1/1 -> If Action Subsystem1/3(pitch_dem)
  PITCHmaxf_1/1 -> If Action Subsystem/2(PITCHmaxf)
  If/3 -> If Action Subsystem2/Action
  PITCHmaxf/1 -> If/2
  Merge/1 -> y/1
  PITCHminf/1 -> If/3
  pitch_dem/1 -> If Action Subsystem/3(pitch_dem)
  If/1 -> If Action Subsystem/Action
  If/2 -> If Action Subsystem1/Action

== system UAV_sync_known_sim_wrong_version/Node 0/VF Approach/BIXLER DYNAMICS/RUBBISH BIN/TECS/PITCH1/integSEB ==
  temp : Inport
  gainInv : Inport  Port=2
  PITCHminf : Inport  Port=3
  PITCHmaxf : Inport  Port=4
  integSEB_delta : Inport  Port=5
  Constant : Constant  Value=0.0783
  Constant1 : Constant  Value=0.0783
  Gain : Gain  Gain=0.1
  Gain1 : Gain  Gain=-0.1
  Product : Product
  Product1 : Product
  Saturation Dynamic : simulink/Discontinuities/Saturation Dynamic  OutMin=[]  OutMax=[]  OutDataTypeStr=Inherit: Same as second input  OutDataType=fixdt(1, 16)  OutScaling=2^-10  DoSatur=off
  Sum{,1,3..4} (4 alike) : Sum  Inputs=|+-
  Sum2 : Sum  Inputs=|++
  gainInv_1 : InportShadow  Port=2
  temp_1 : InportShadow
  "IntegSEB_delta " : Outport
  "integSEB_min " : Outport  Port=2
  integSEB_max : Outport  Port=3
  wires:
  PITCHminf/1 -> Sum/1
  Product/1 -> Sum1/1
  Constant1/1 -> Sum2/2
  Sum3/1 -> integSEB_max/1, [integSEB_max]
  PITCHmaxf/1 -> Sum2/1
  Sum2/1 -> Product1/2
  Product1/1 -> Sum3/1
  gainInv_1/1 -> Product1/1
  temp_1/1 -> Sum3/2
  Constant/1 -> Sum/2
  integSEB_delta/1 -> Saturation Dynamic/2
  Sum/1 -> Product/2
  Sum1/1 -> "integSEB_min "/1, [integSEB_min]
  temp/1 -> Sum1/2
  [integSEB_range] -> Gain1/1
  Gain1/1 -> Saturation Dynamic/3
  Saturation Dynamic/1 -> "IntegSEB_delta "/1
  Sum4/1 -> [integSEB_range]
  [integSEB_min] -> Sum4/2
  [integSEB_max] -> Sum4/1
  [integSEB_range] -> Gain/1
  Gain/1 -> Saturation Dynamic/1
  gainInv/1 -> Product/1

== system UAV_sync_known_sim_wrong_version/Node 0/VF Approach/BIXLER DYNAMICS/RUBBISH BIN/TECS/PITCH1/timeConstant() ==
  Constant1 : Constant  Value=0.1
  Constant5 : Constant  Value=Ctr.TECS.TIME_CONST
  MinMax : MinMax  Function=max  Inputs=2
  timeConstant : Outport
  wires:
  MinMax/1 -> timeConstant/1
  Constant1/1 -> MinMax/2
  Constant5/1 -> MinMax/1

== system UAV_sync_known_sim_wrong_version/Node 0/VF Approach/BIXLER DYNAMICS/RUBBISH BIN/TECS/PITCH1/timeConstant()1 ==
  Constant1 : Constant  Value=0.1
  Constant5 : Constant  Value=Ctr.TECS.TIME_CONST
  MinMax : MinMax  Function=max  Inputs=2
  timeConstant : Outport
  wires:
  MinMax/1 -> timeConstant/1
  Constant1/1 -> MinMax/2
  Constant5/1 -> MinMax/1

== system UAV_sync_known_sim_wrong_version/Node 0/VF Approach/BIXLER DYNAMICS/Vehicle Airframe/Aerodynamics/Aerodynamic Coefficients/Forces ==
  note: CL
  note: Cy
  note: CD
  note: f_y is already in the body frame
  alpha_k : Inport
  alpha_f : Inport  Port=2
  CD interpolation : Interpolation_n-D  NumberOfTableDimensions=1  Table=Aero.CD_Basic  RemoveProtectionIndex=on  InternalRulePriority=Speed
      settings: InputPortMap=u0,u1
  CL interpolation : Interpolation_n-D  NumberOfTableDimensions=1  Table=Aero.CL_Basic  RemoveProtectionIndex=on  InternalRulePriority=Speed
      settings: InputPortMap=u0,u1
  CYp Interpolation : Interpolation_n-D  NumberOfTableDimensions=1  Table=Aero.Cy_RollRate  RemoveProtectionIndex=on  InternalRulePriority=Speed
      settings: InputPortMap=u0,u1
  Constant1 : Constant  Value=Aero.CL_PitchRate
  Constant6 : Constant  Value=Aero.Cy_Beta
  Divide1 : Product  Inputs=**/
  Divide3 : Product  Inputs=**
  Divide4 : Product  Inputs=**/
  Gain10 : Gain  Gain=2
  Gain2 : Gain  Gain=Bxl.c
  Gain3 : Gain  Gain=2
  Gain9 : Gain  Gain=Bxl.b
  Sum1 : Sum  Inputs=|++
  Sum3 : Sum  Inputs=++|
  CD : Outport
  Cy : Outport  Port=2
  CL : Outport  Port=3
  wires:
  Gain2/1 -> Divide1/1
  Constant1/1 -> Gain2/1
  Gain3/1 -> Divide1/3
  [Va] -> Gain3/1
  [qRad] -> Divide1/2  "q=pitch rate"
  Divide1/1 -> Sum1/2
  [pRad] -> Divide4/2  "q=roll rate"
  [Va] -> Gain10/1
  Gain9/1 -> Divide4/1
  Gain10/1 -> Divide4/3
  Sum3/1 -> Cy/1  "Cy"
  CL interpolation/1 -> Sum1/1  "CL(alpha)"
  CYp Interpolation/1 -> Gain9/1
  alpha_k/1 -> CL interpolation/1, CYp Interpolation/1, CD interpolation/1
  alpha_f/1 -> CL interpolation/2, CYp Interpolation/2, CD interpolation/2
  Divide4/1 -> Sum3/2
  CD interpolation/1 -> CD/1  "CD(alpha)"
  Sum1/1 -> CL/1  "CL"
  [BetaRad] -> Divide3/2
  Constant6/1 -> Divide3/1
  Divide3/1 -> Sum3/1

== system UAV_sync_known_sim_wrong_version/Node 0/VF Approach/BIXLER DYNAMICS/Vehicle Airframe/Aerodynamics/Aerodynamic Coefficients/Moments ==
  note: Cn
  note: Cl
  note: Cm
  note: Moments already in the body frame
  alpha_k : Inport
  alpha_f : Inport  Port=2
  Clb Interpolation : Interpolation_n-D  NumberOfTableDimensions=1  Table=Aero.Cl_Beta  RemoveProtectionIndex=on  InternalRulePriority=Speed
      settings: InputPortMap=u0,u1
  Clp Interpolation : Interpolation_n-D  NumberOfTableDimensions=1  Table=Aero.Cl_RollRate  RemoveProtectionIndex=on  InternalRulePriority=Speed
      settings: InputPortMap=u0,u1
  Clr Interpolation : Interpolation_n-D  NumberOfTableDimensions=1  Table=Aero.Cl_YawRate  RemoveProtectionIndex=on  InternalRulePriority=Speed
      settings: InputPortMap=u0,u1
  Cm_Basic Interpolation : Interpolation_n-D  NumberOfTableDimensions=1  Table=Aero.Cm_Basic  RemoveProtectionIndex=on  InternalRulePriority=Speed
      settings: InputPortMap=u0,u1
  Cnp : Interpolation_n-D  NumberOfTableDimensions=1  Table=Aero.Cn_RollRate  RemoveProtectionIndex=on  InternalRulePriority=Speed
      settings: InputPortMap=u0,u1
  Cnr : Interpolation_n-D  NumberOfTableDimensions=1  Table=Aero.Cn_YawRate  RemoveProtectionIndex=on  InternalRulePriority=Speed
      settings: InputPortMap=u0,u1
  Constant1 : Constant  Value=0
  Constant2 : Constant  Value=Aero.Cm_PitchRate
  Constant4 : Constant  Value=0
  Constant5 : Constant  Value=Aero.Cn_Beta
  Divide1 : Product  Inputs=**
  Divide3 : Product  Inputs=**
  Divide{4..7,9} (5 alike) : Product  Inputs=**/
  Gain{1,3..4,7,15} (5 alike) : Gain  Gain=2
  Gain{2,5,8,13} (4 alike) : Gain  Gain=Bxl.b
  Gain14 : Gain  Gain=Bxl.c
  Manual Switch2 : ManualSwitch
  Manual Switch3 : ManualSwitch
  Sum{1..2,4..5} (4 alike) : Sum  Inputs=|++
  Sum3 : Sum  Inputs=++|
  Cl : Outport
  Cm : Outport  Port=2
  Cn : Outport  Port=3
  wires:
  alpha_k/1 -> Cnr/1, Cnp/1, Cm_Basic Interpolation/1, Clr Interpolation/1, Clp Interpolation/1, Clb Interpolation/1
  alpha_f/1 -> Cnr/2, Cnp/2, Cm_Basic Interpolation/2, Clr Interpolation/2, Clp Interpolation/2, Clb Interpolation/2
  [Va] -> Gain3/1
  Divide9/1 -> Sum1/2
  Sum1/1 -> Sum3/2
  Gain1/1 -> Divide9/3
  [Va] -> Gain1/1
  Gain2/1 -> Divide9/1
  [rRad] -> Divide9/2  "r=yaw rate"
  Cnp/1 -> Gain8/1
  [pRad] -> Divide4/2  "p=roll rate"
  Sum3/1 -> Cn/1  "Cn"
  Gain8/1 -> Divide4/1
  Gain3/1 -> Divide4/3
  Cnr/1 -> Gain2/1
  Divide3/1 -> Sum2/1
  Clb Interpolation/1 -> Divide3/1
  Gain7/1 -> Divide6/3
  [Va] -> Gain4/1
  Gain4/1 -> Divide5/3
  Sum4/1 -> Cl/1  "Cl"
  Gain5/1 -> Divide5/1
  Gain13/1 -> Divide6/1
  Clp Interpolation/1 -> Gain5/1
  [BetaRad] -> Divide3/2
  [Va] -> Gain7/1
  Clr Interpolation/1 -> Gain13/1
  Divide6/1 -> Manual Switch2/1
  [pRad] -> Divide5/2  "p=roll rate"
  Sum2/1 -> Sum4/1
  [rRad] -> Divide6/2  "r=yaw rate"
  [qRad] -> Divide7/2  "q=pitch rate"
  Gain15/1 -> Divide7/3
  Gain14/1 -> Divide7/1
  Sum5/1 -> Cm/1  "Cm"
  Constant2/1 -> Gain14/1
  Cm_Basic Interpolation/1 -> Sum5/1
  [Va] -> Gain15/1
  Divide7/1 -> Sum5/2
  Divide1/1 -> Sum3/1
  [BetaRad] -> Divide1/2
  Constant5/1 -> Divide1/1
  Divide4/1 -> Sum1/1
  Constant4/1 -> Manual Switch3/2
  Divide5/1 -> Manual Switch3/1
  Manual Switch3/1 -> Sum2/2
  Manual Switch2/1 -> Sum4/2
  Constant1/1 -> Manual Switch2/2

== system UAV_sync_known_sim_wrong_version/Node 0/VF Approach/BIXLER DYNAMICS/Vehicle Airframe/Aerodynamics/ControlIncrements/Ailerons ==
  alpha_k : Inport
  alpha_f : Inport  Port=2
  DeltaAil : Inport  Port=3
  Cl_ail Interpolation : Interpolation_n-D  NumberOfTableDimensions=1  Table=Aero.Cl_ail  RemoveProtectionIndex=on  InternalRulePriority=Speed
      settings: InputPortMap=u0,u1
  Cn_ail Interpolation : Interpolation_n-D  Table=Aero.Cn_ail  InternalRulePriority=Speed
  DeltaAil. : PreLookup  BreakpointsData=Aero.delta_ail_vector  BeginIndexSearchUsingPreviousIndexResult=on  ExtrapMethod=Linear  RemoveProtectionInput=on
  Cn_ail : Outport
  Cl_ail : Outport  Port=2
  wires:
  DeltaAil/1 -> DeltaAil./1
  Cn_ail Interpolation/1 -> Cn_ail/1
  Cl_ail Interpolation/1 -> Cl_ail/1
  alpha_f/1 -> Cn_ail Interpolation/2
  DeltaAil./2 -> Cl_ail Interpolation/2, Cn_ail Interpolation/4
  DeltaAil./1 -> Cl_ail Interpolation/1, Cn_ail Interpolation/3
  alpha_k/1 -> Cn_ail Interpolation/1

== system UAV_sync_known_sim_wrong_version/Node 0/VF Approach/BIXLER DYNAMICS/Vehicle Airframe/Aerodynamics/ControlIncrements/Elevator ==
  alpha_k : Inport
  alpha_f : Inport  Port=2
  DeltaElev : Inport  Port=3
  CD_elev Interpolation : Interpolation_n-D  Table=Aero.CD_elev  RemoveProtectionIndex=on  InternalRulePriority=Speed
  DeltaElev Interpolation : PreLookup  BreakpointsData=Aero.delta_ail_vector  BeginIndexSearchUsingPreviousIndexResult=on  ExtrapMethod=Linear  RemoveProtectionInput=on
  Gain : Gain  Gain=Aero.CL_elev
  Gain1 : Gain  Gain=Aero.Cm_elev
  Scope : Scope
  Scope1 : Scope
  CD_elev : Outport
  CL_elev : Outport  Port=2
  Cm_elev : Outport  Port=3
  wires:
  Gain1/1 -> Scope1/1, Cm_elev/1
  DeltaElev/1 -> DeltaElev Interpolation/1, Gain1/1, Gain/1
  alpha_k/1 -> CD_elev Interpolation/1
  DeltaElev Interpolation/1 -> CD_elev Interpolation/3
  DeltaElev Interpolation/2 -> CD_elev Interpolation/4
  alpha_f/1 -> CD_elev Interpolation/2
  CD_elev Interpolation/1 -> Scope/1, CD_elev/1
  Gain/1 -> CL_elev/1

== system UAV_sync_known_sim_wrong_version/Node 0/VF Approach/BIXLER DYNAMICS/Vehicle Airframe/Aerodynamics/ControlIncrements/Rudder ==
  note: Change of sign to match with the convention.
      | The coefficients are taken from a report of the Bixler 2 flight.
  deltaRudd : Inport
  Gain : Gain  Gain=-1
  Gain1 : Gain  Gain=Aero.Cy_rudd
  Gain2 : Gain  Gain=Aero.Cn_rudd
  Gain3 : Gain  Gain=Aero.Cl_rudd
  Gain4 : Gain  Gain=-1
  Cy_rudd : Outport
  Cl_rudd : Outport  Port=2
  Cn_rudd : Outport  Port=3
  wires:
  Gain3/1 -> Gain4/1
  Gain1/1 -> Gain/1
  deltaRudd/1 -> Gain1/1, Gain3/1, Gain2/1
  Gain2/1 -> Cn_rudd/1
  Gain4/1 -> Cl_rudd/1
  Gain/1 -> Cy_rudd/1

== system UAV_sync_known_sim_wrong_version/Node 0/VF Approach/AUTOPILOT/Low-level Controllers/Pitch controller/Pitch PID/Anti-windup/If Action Subsystem ==
  In1 : Inport
  Action Port : ActionPort  ActionType=then
  Constant : Constant  Value=0
  MinMax : MinMax  Function=max  Inputs=2
  Out1 : Outport
  wires:
  In1/1 -> MinMax/1
  Constant/1 -> MinMax/2
  MinMax/1 -> Out1/1

== system UAV_sync_known_sim_wrong_version/Node 0/VF Approach/AUTOPILOT/Low-level Controllers/Pitch controller/Pitch PID/Anti-windup/If Action Subsystem1 ==
  In1 : Inport
  Action Port : ActionPort  ActionType=elseif
  Constant : Constant  Value=0
  MinMax : MinMax  Inputs=2
  Out1 : Outport
  wires:
  In1/1 -> MinMax/1
  Constant/1 -> MinMax/2
  MinMax/1 -> Out1/1

== system UAV_sync_known_sim_wrong_version/Node 0/VF Approach/AUTOPILOT/Low-level Controllers/Pitch controller/Pitch PID/Anti-windup/If Action Subsystem2 ==
  In1 : Inport
  Action Port : ActionPort  ActionType=else
  Out1 : Outport
  wires:
  In1/1 -> Out1/1

== system UAV_sync_known_sim_wrong_version/Node 0/VF Approach/AUTOPILOT/Low-level Controllers/Pitch controller/Pitch PID/Subsystem/If Action Subsystem ==
  In1 : Inport
  Action Port : ActionPort
  Constant : Constant  Value=180
  Sum : Sum  Inputs=|+-
  Out1 : Outport
  wires:
  In1/1 -> Sum/2
  Constant/1 -> Sum/1
  Sum/1 -> Out1/1

== system UAV_sync_known_sim_wrong_version/Node 0/VF Approach/AUTOPILOT/Low-level Controllers/Pitch controller/Pitch PID/Subsystem/If Action Subsystem1 ==
  In1 : Inport
  Action Port : ActionPort
  Out1 : Outport
  wires:
  In1/1 -> Out1/1

== system UAV_sync_known_sim_wrong_version/Node 0/VF Approach/AUTOPILOT/Low-level Controllers/Pitch controller/Pitch PID/Subsystem/If Action Subsystem2 ==
  In1 : Inport
  In2 : Inport  Port=2
  Action Port : ActionPort
  Fcn : Fcn  Expr=1- ((u(1)-(APlane.roll_limit+5))/(90-APlane.roll_limit))
  Product7 : Product
  Out1 : Outport
  wires:
  In1/1 -> Fcn/1
  Fcn/1 -> Product7/1
  Product7/1 -> Out1/1
  In2/1 -> Product7/2

== system UAV_sync_known_sim_wrong_version/Node 0/VF Approach/AUTOPILOT/Low-level Controllers/Pitch controller/Pitch PID/Subsystem/If Action Subsystem3 ==
  In1 : Inport
  Action Port : ActionPort
  Out1 : Outport
  wires:
  In1/1 -> Out1/1

== system UAV_sync_known_sim_wrong_version/Node 0/VF Approach/AUTOPILOT/Low-level Controllers/Pitch controller/TRASH/If Action Subsystem1/cosd ==
  In1 : Inport
  Angle Conversion : aerolibconvert2/Angle Conversion  IU=deg  OU=rad
  Angle Conversion1 : aerolibconvert2/Angle Conversion  IU=rad  OU=deg
  Trigonometric Function : Trigonometry  Operator=cos
  Out1 : Outport
  wires:
  Trigonometric Function/1 -> Angle Conversion1/1
  Angle Conversion/1 -> Trigonometric Function/1
  Angle Conversion1/1 -> Out1/1
  In1/1 -> Angle Conversion/1

== system UAV_sync_known_sim_wrong_version/Node 0/VF Approach/AUTOPILOT/Low-level Controllers/Pitch controller/TRASH/If Action Subsystem1/sind ==
  In1 : Inport
  Angle Conversion : aerolibconvert2/Angle Conversion  IU=deg  OU=rad
  Angle Conversion1 : aerolibconvert2/Angle Conversion  IU=rad  OU=deg
  Trigonometric Function : Trigonometry
  Out1 : Outport
  wires:
  Trigonometric Function/1 -> Angle Conversion1/1
  Angle Conversion/1 -> Trigonometric Function/1
  Angle Conversion1/1 -> Out1/1
  In1/1 -> Angle Conversion/1

== system UAV_sync_known_sim_wrong_version/Node 0/VF Approach/AUTOPILOT/Low-level Controllers/Pitch controller/TRASH/If Action Subsystem1/tand ==
  In1 : Inport
  Angle Conversion : aerolibconvert2/Angle Conversion  IU=deg  OU=rad
  Angle Conversion1 : aerolibconvert2/Angle Conversion  IU=rad  OU=deg
  Trigonometric Function : Trigonometry  Operator=tan
  Out1 : Outport
  wires:
  In1/1 -> Angle Conversion/1
  Angle Conversion1/1 -> Out1/1
  Angle Conversion/1 -> Trigonometric Function/1
  Trigonometric Function/1 -> Angle Conversion1/1

== system UAV_sync_known_sim_wrong_version/Node 0/VF Approach/AUTOPILOT/Low-level Controllers/Roll controller/Roll Rate Controller/Anti-windup/If Action Subsystem ==
  In1 : Inport
  Action Port : ActionPort  ActionType=then
  Constant : Constant  Value=0
  MinMax : MinMax  Function=max  Inputs=2
  Out1 : Outport
  wires:
  In1/1 -> MinMax/1
  Constant/1 -> MinMax/2
  MinMax/1 -> Out1/1

== system UAV_sync_known_sim_wrong_version/Node 0/VF Approach/AUTOPILOT/Low-level Controllers/Roll controller/Roll Rate Controller/Anti-windup/If Action Subsystem1 ==
  In1 : Inport
  Action Port : ActionPort  ActionType=elseif
  Constant : Constant  Value=0
  MinMax : MinMax  Inputs=2
  Out1 : Outport
  wires:
  In1/1 -> MinMax/1
  Constant/1 -> MinMax/2
  MinMax/1 -> Out1/1

== system UAV_sync_known_sim_wrong_version/Node 0/VF Approach/AUTOPILOT/Low-level Controllers/Roll controller/Roll Rate Controller/Anti-windup/If Action Subsystem2 ==
  In1 : Inport
  Action Port : ActionPort  ActionType=else
  Out1 : Outport
  wires:
  In1/1 -> Out1/1

== system UAV_sync_known_sim_wrong_version/Node 0/VF Approach/BIXLER DYNAMICS/RUBBISH BIN/TECS/PITCH/Limiter/If Action Subsystem ==
  integSEB_input : Inport
  PITCHmaxf : Inport  Port=2
  pitch_dem : Inport  Port=3
  Action Port : ActionPort
  MinMax : MinMax
  Mux : Mux  Inputs=2
  Sum : Sum  Inputs=|+-
  Out1 : Outport
  wires:
  integSEB_input/1 -> Mux/1
  MinMax/1 -> Out1/1
  PITCHmaxf/1 -> Sum/1
  Sum/1 -> Mux/2
  Mux/1 -> MinMax/1
  pitch_dem/1 -> Sum/2

== system UAV_sync_known_sim_wrong_version/Node 0/VF Approach/BIXLER DYNAMICS/RUBBISH BIN/TECS/PITCH/Limiter/If Action Subsystem1 ==
  integSEB_input : Inport
  PITCHminf : Inport  Port=2
  pitch_dem : Inport  Port=3
  Action Port : ActionPort
  MinMax : MinMax  Function=max
  Mux : Mux  Inputs=2
  Sum : Sum  Inputs=|+-
  Out1 : Outport
  wires:
  integSEB_input/1 -> Mux/1
  MinMax/1 -> Out1/1
  PITCHminf/1 -> Sum/1
  pitch_dem/1 -> Sum/2
  Sum/1 -> Mux/2
  Mux/1 -> MinMax/1

== system UAV_sync_known_sim_wrong_version/Node 0/VF Approach/BIXLER DYNAMICS/RUBBISH BIN/TECS/PITCH/Limiter/If Action Subsystem2 ==
  integSEB_input : Inport
  Action Port : ActionPort
  Out1 : Outport
  wires:
  integSEB_input/1 -> Out1/1

== system UAV_sync_known_sim_wrong_version/Node 0/VF Approach/BIXLER DYNAMICS/RUBBISH BIN/TECS/PITCH1/Limiter/If Action Subsystem ==
  integSEB_input : Inport
  PITCHmaxf : Inport  Port=2
  pitch_dem : Inport  Port=3
  Action Port : ActionPort
  MinMax : MinMax
  Mux : Mux  Inputs=2
  Sum : Sum  Inputs=|+-
  Out1 : Outport
  wires:
  integSEB_input/1 -> Mux/1
  MinMax/1 -> Out1/1
  PITCHmaxf/1 -> Sum/1
  Sum/1 -> Mux/2
  Mux/1 -> MinMax/1
  pitch_dem/1 -> Sum/2

== system UAV_sync_known_sim_wrong_version/Node 0/VF Approach/BIXLER DYNAMICS/RUBBISH BIN/TECS/PITCH1/Limiter/If Action Subsystem1 ==
  integSEB_input : Inport
  PITCHminf : Inport  Port=2
  pitch_dem : Inport  Port=3
  Action Port : ActionPort
  MinMax : MinMax  Function=max
  Mux : Mux  Inputs=2
  Sum : Sum  Inputs=|+-
  Out1 : Outport
  wires:
  integSEB_input/1 -> Mux/1
  MinMax/1 -> Out1/1
  PITCHminf/1 -> Sum/1
  pitch_dem/1 -> Sum/2
  Sum/1 -> Mux/2
  Mux/1 -> MinMax/1

== system UAV_sync_known_sim_wrong_version/Node 0/VF Approach/BIXLER DYNAMICS/RUBBISH BIN/TECS/PITCH1/Limiter/If Action Subsystem2 ==
  integSEB_input : Inport
  Action Port : ActionPort
  Out1 : Outport
  wires:
  integSEB_input/1 -> Out1/1

== matlab function UAV_sync_known_sim_wrong_version/Node 0/VF Approach/BIXLER DYNAMICS/RUBBISH BIN/Orbit/Loiter Controller/Beard Version ==
  data: chi input; chi_c output; chi_d input; d input; Vg input; gamma input; param input
function chi_c  = OrbitController(chi, chi_d, d, Vg, gamma, param)

%%
k = param(1);
kk = param(2);
epsi = param(3);
r = param(4);
j = param(5);
alpha = param(6);

%%
chi_tilde = chi-chi_d;
lt = chi_tilde/epsi;

if abs(lt) <=1
    term = lt;
else
    term = sign(lt);
end

d_tilde = d-r;
beta = k/(1+(k*d_tilde)^2);

err = (chi-gamma);

term2 = Vg /(alpha*d)*sin(err) + j*beta/alpha*Vg*cos(err);

term3 = -kk/alpha*term;

chi_c = chi + term2 + term3;
